simulink model "Engine_MC_Wit_System1"  (R2014b)
settings: Solver=ode15s  StartTime=0.0  StopTime=100  RelTol=1e-3
undefined symbols (not defined in the file): sigbuilder_block
libraries: fl_lib x19, nesl_utility x9, sdl_lib x4, simulink x4
settings Model: Creator=wnursilo  LastModifiedBy=wnursilo
settings SolverCC: ZeroCrossAlgorithm=Adaptive
settings SimscapeCC: SimscapeLogType=local  SimscapeLogLimitData=off

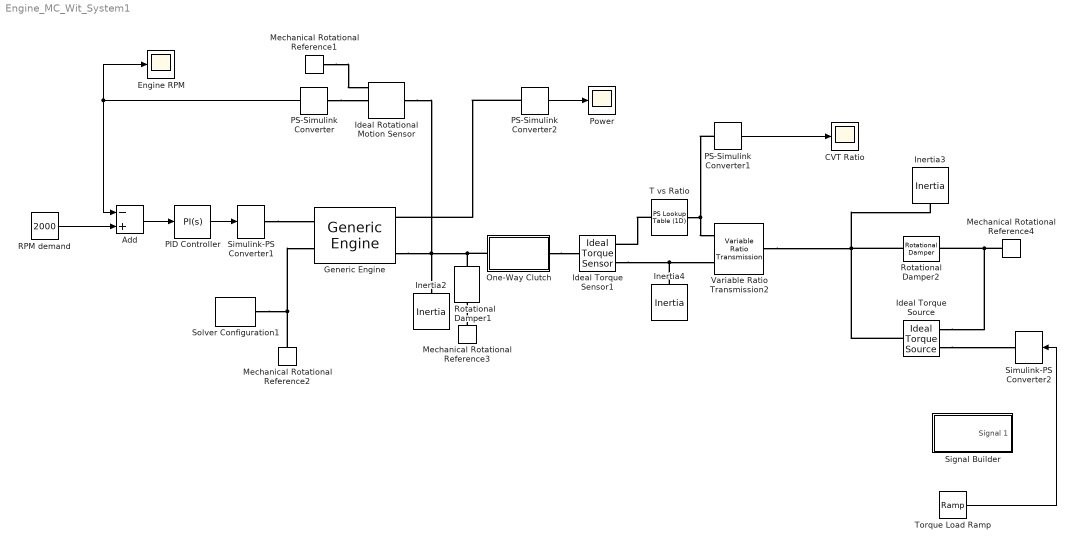
== system Engine_MC_Wit_System1 ==
  Add : Sum  Inputs=-+
  CVT Ratio : Scope
      settings: YMin=3  YMax=11
  Engine RPM : Scope
      settings: YMin=750  YMax=2750
  Generic Engine : sdl_lib/Engines/Generic Engine  model_parameterization=1  engine_type=1  P_max=8300 W  w_P_max=8500 rpm  w_max=9000 rpm  w_min=500 rpm  w_tab=[ 500 1000 2e+3 3e+3 4e+3 5e+3 6e+3 7e+3 ] rpm  trq_tab=[ 380 380 380 380 350 280 200 80 ] N*m  pwr_tab=[ 2e+4 4e+4 7.8e+4 1.2e+5 1.45e+5 1.48e+5 1.25e+5 6e+4 ] W  interp_method=1  model_inertia=0  inertia=1 kg*m^2  initial_velocity=800 rpm  model_time_constant=0  time_constant=0.2 s  T0=0  w_thr=100 rpm  idle_speed=0  idle_speed_reference=1000 rpm  tau_controller=0.1 s  idle_w_thr=10 rpm  fc_model=1  fc_per_rev=25 mg/rev  displaced_volume=400 cm^3  rev_per_cycle=2  fc_w_tab=[ 1000 2e+3 3e+3 4e+3 5e+3 6e+3 ] rpm  fc_trq_tab=[ 0 80 160 200 240 320 360 400 ] N*m  fc_tab=[ 0.5 0.9 1.4 1.6 1.9 2.7 3.4 4.4; 1 1.7 2.7 3.1 3.6 5 6 7.4; 1.4 2.7 4 4.8 5.6 7.5 8.5 10.5; 2 3.6 5.8 6.7 8 10.4 11.7 13.3; 2.5 4.8 7.9 9.4 10.8 14 16.2 18.6; 3.1 6 10.3 11.9 13.8 18.4 22 26.5 ] g/s  bmep_tab=[ 0 250 500 625 750 1000 1.15e+3 1.25e+3 ] kPa  bsfc_tab=[ 410 380 300 280 270 290 320 380; 410 370 290 270 260 270 285 320; 415 380 290 275 265 270 270 300; 420 390 310 290 285 280 280 285; 430 410 340 320 310 300 310 320; 450 430 370 340 330 330 350 380 ] g/hr/kW  fc_interp_method=1
  Ideal Rotational Motion Sensor : fl_lib/Mechanical/Mechanical Sensors/Ideal Rotational Motion Sensor  offset=0 rad
  Ideal Torque Sensor1 : fl_lib/Mechanical/Mechanical Sensors/Ideal Torque Sensor
  Ideal Torque Source : fl_lib/Mechanical/Mechanical Sources/Ideal Torque Source
  Inertia2 : fl_lib/Mechanical/Rotational Elements/Inertia  inertia=HEV_Param.ICE.Shaft_Inertia kg*m^2  w_specify=on  w_priority=High  w=800 rpm  t_specify=off  t_priority=High  t=0 N*m
  Inertia3 : fl_lib/Mechanical/Rotational Elements/Inertia  inertia=HEV_Param.ICE.Shaft_Inertia kg*m^2  w_specify=on  w_priority=Low  w=0 rad/s  t_specify=off  t_priority=High  t=0 N*m
      settings: LogSimulationData=on
  Inertia4 : fl_lib/Mechanical/Rotational Elements/Inertia  inertia=HEV_Param.ICE.Shaft_Inertia kg*m^2  w_specify=on  w_priority=Low  w=0 rpm  t_specify=off  t_priority=High  t=0 N*m
  Mechanical Rotational Reference{1..4} (4 alike) : fl_lib/Mechanical/Rotational Elements/Mechanical Rotational Reference
  One-Way Clutch : Subsystem
  PID Controller : simulink/Continuous/PID Controller  Controller=PI  TimeDomain=Continuous-time  SampleTime=-1  IntegratorMethod=Forward Euler  FilterMethod=Forward Euler  Form=Parallel  P=10  I=1  D=0  N=100  InitialConditionSource=internal  InitialConditionForIntegrator=0  InitialConditionForFilter=0  ExternalReset=none  LimitOutput=off  UpperSaturationLimit=inf  LowerSaturationLimit=-inf  LinearizeAsGain=on  AntiWindupMode=none  Kb=1  TrackingMode=off  Kt=1  PParamMin=[]  PParamMax=[]  IParamMin=[]  IParamMax=[]  DParamMin=[]  DParamMax=[]  NParamMin=[]  NParamMax=[]  KbParamMin=[]  KbParamMax=[]  KtParamMin=[]  KtParamMax=[]  POutMin=[]  POutMax=[]  IOutMin=[]  IOutMax=[]  DOutMin=[]  DOutMax=[]  NOutMin=[]  NOutMax=[]  KbOutMin=[]  KbOutMax=[]  KtOutMin=[]  KtOutMax=[]  IntegratorOutMin=[]  IntegratorOutMax=[]  FilterOutMin=[]  FilterOutMax=[]  SumOutMin=[]  SumOutMax=[]  SumI1OutMin=[]  SumI1OutMax=[]  SumI2OutMin=[]  SumI2OutMax=[]  SumI3OutMin=[]  SumI3OutMax=[]  SumDOutMin=[]  SumDOutMax=[]  SaturationOutMin=[]  SaturationOutMax=[]  IntegratorContinuousStateAttributes=''  IntegratorStateMustResolveToSignalObject=off  IntegratorRTWStateStorageClass=Auto  FilterContinuousStateAttributes=''  FilterStateMustResolveToSignalObject=off  FilterRTWStateStorageClass=Auto  DifferentiatorICPrevScaledInput=0  DifferentiatorOutMin=[]  DifferentiatorOutMax=[]  UseFilter=on
  PS-Simulink Converter : nesl_utility/PS-Simulink Converter  PhysicalDomain=network_engine_domain  SubClassName=ps_output  LeftPortType=input  RightPortType=output  PseudoPeriodic=off  Frequencies=[]  Unit=rpm  AffineConversion=off
  PS-Simulink Converter1 : nesl_utility/PS-Simulink Converter  PhysicalDomain=network_engine_domain  SubClassName=ps_output  LeftPortType=input  RightPortType=output  PseudoPeriodic=off  Frequencies=[]  Unit=1  AffineConversion=off
  PS-Simulink Converter2 : nesl_utility/PS-Simulink Converter  PhysicalDomain=network_engine_domain  SubClassName=ps_output  LeftPortType=input  RightPortType=output  PseudoPeriodic=off  Frequencies=[]  Unit=1  AffineConversion=off
  Power : Scope
      settings: YMin=5250  YMax=7500  SaveName=ScopeData3
  RPM demand : Constant  Value=2000
  Rotational Damper1 : fl_lib/Mechanical/Rotational Elements/Rotational Damper  D=0.01 N*m/(rad/s)  w_specify=off  w_priority=High  w=0 rad/s  t_specify=off  t_priority=High  t=0 N*m
  Rotational Damper2 : fl_lib/Mechanical/Rotational Elements/Rotational Damper  D=0.001 N*m/(rad/s)  w_specify=off  w_priority=High  w=0 rad/s  t_specify=off  t_priority=High  t=0 N*m
  Signal Builder : Subsystem  Tag=STV Subsys  LoadFcn=sigbuilder_block('load');  StartFcn=sigbuilder_block('start');  StopFcn=sigbuilder_block('stop');  ClipboardFcn=sigbuilder_block('clipboard');  mask(Sigbuilder block){}
      mask help: Simulink:masks:SigbuilderBlock_MD
      mask init:
      | if ~strcmp(get_param(bdroot(gcbh),'SimulationStatus'),'stopped') tuvar = sigbuilder_block('maskInit'); end
      settings: CopyFcn=sigbuilder_block('copy');  DeleteFcn=sigbuilder_block('delete');  ModelCloseFcn=sigbuilder_block('modelClose');  PreSaveFcn=sigbuilder_block('preSave');  PauseFcn=sigbuilder_block('pause');  ContinueFcn=sigbuilder_block('continue');  NameChangeFcn=sigbuilder_block('namechange');  OpenFcn=sigbuilder_block('open',[437.25 199.5 550.5 399.75 ]);  CloseFcn=sigbuilder_block('close');
      mask Display: plot(0, 0, 100, 100,[2, 2, 32, 32, 2], [68, 8, 8, 68, 68],[32, 2], [38, 38], [32, 19, 2],[53, 60, 44], [32, 17, 17, 2],[16, 16, 31, 31]);txt = getActiveGroup(gcbh);text(2, 100, txt,'verticalAlignment', 'top');
  Simulink-PS Converter1 : nesl_utility/Simulink-PS Converter  PhysicalDomain=network_engine_domain  SubClassName=ps_input  LeftPortType=input  RightPortType=output  PseudoPeriodic=off  Frequencies=[]  NoiseDistribution=none  NoiseParameters=[]  Unit=1  AffineConversion=off  InputFiltering=on  SimscapeFilterOrder=1  InputFilterTimeConstant=0.001  UdotUserProvided=1
  Simulink-PS Converter2 : nesl_utility/Simulink-PS Converter  PhysicalDomain=network_engine_domain  SubClassName=ps_input  LeftPortType=input  RightPortType=output  PseudoPeriodic=off  Frequencies=[]  NoiseDistribution=none  NoiseParameters=[]  Unit=1  AffineConversion=off  InputFiltering=off  SimscapeFilterOrder=1  InputFilterTimeConstant=0.001  UdotUserProvided=1
  Solver Configuration1 : nesl_utility/Solver Configuration  PhysicalDomain=network_engine_domain  SubClassName=solver  LeftPortType=input  RightPortType=generic  Accelerate=off  Tones=[]  Harmonics=[]  SimulateNoise=off  Profile=off  UseLocalSampling=off  EnableSwitchedLinearOptims=on  FrequencyDomain=off  UseCCode=off  RelTol=0.001  AbsTol=1e-06  MinStep=1e-09  ToWorkspace=off  DoDC=off  ResidualTolerance=1e-09  UseLocalSolver=off  LocalSolverChoice=NE_BACKWARD_EULER_ADVANCER  LocalSolverSampleTime=0.001  DoFixedCost=off  MaxNonlinIter=3  MaxModeIter=2  LinearAlgebra=Sparse  DelaysMemoryBudget=1024  AutomaticFiltering=on  FilteringTimeConstant=0.001
  T vs Ratio : fl_lib/Physical Signals/Lookup Tables/PS Lookup Table (1D)  x_t="[1e3, 100,  80, 60, 40, 20, 10, 8, 6, 4, 2, 0]"  y_t=[10, 10, 8, 6, 4, 2, 1, 0.8, 0.6, 0.4, 0.2, 0.2]  interp_method=1  extrap_method=2
  Torque Load Ramp : simulink/Sources/Ramp  slope=-10  start=2  X0=0
  Variable Ratio Transmission2 : sdl_lib/Couplings & Drives/Variable Ratio Transmission  rotation_direction=1  kp=3e+5 N*m/rad  kv=100 N*m/(rad/s)  initial_torque=0 N*m  losses_model=1  efficiency=0.8  mu_visc=[ 0 0 ] N*m/(rad/s)  w_thr=0.01 rad/s
  wires:
  RPM demand/1 -> Add/2
  PS-Simulink Converter/1 -> Engine RPM/1, Add/1
  Add/1 -> PID Controller/1
  PID Controller/1 -> Simulink-PS Converter1/1
  Torque Load Ramp/1 -> Simulink-PS Converter2/1
  PS-Simulink Converter1/1 -> CVT Ratio/1
  PS-Simulink Converter2/1 -> Power/1
  connections:
  Mechanical Rotational Reference2/LConn1 -- Solver Configuration1/RConn1 -- Generic Engine/LConn2
  Generic Engine/RConn3 -- One-Way Clutch/LConn1 -- Rotational Damper1/LConn1 -- Ideal Rotational Motion Sensor/LConn1 -- Inertia2/LConn1
  Simulink-PS Converter1/RConn1 -- Generic Engine/LConn1
  Mechanical Rotational Reference3/LConn1 -- Rotational Damper1/RConn1
  Rotational Damper2/LConn1 -- Ideal Torque Source/LConn1 -- Inertia3/LConn1 -- Variable Ratio Transmission2/RConn1
  Mechanical Rotational Reference4/LConn1 -- Ideal Torque Source/RConn2 -- Rotational Damper2/RConn1
  One-Way Clutch/RConn1 -- Ideal Torque Sensor1/LConn1
  Ideal Torque Sensor1/RConn1 -- Inertia4/LConn1 -- Variable Ratio Transmission2/LConn2
  T vs Ratio/LConn1 -- Ideal Torque Sensor1/RConn2
  T vs Ratio/RConn1 -- Variable Ratio Transmission2/LConn1 -- PS-Simulink Converter1/LConn1
  PS-Simulink Converter/LConn1 -- Ideal Rotational Motion Sensor/RConn2
  Mechanical Rotational Reference1/LConn1 -- Ideal Rotational Motion Sensor/RConn1
  Ideal Torque Source/RConn1 -- Simulink-PS Converter2/RConn1
  PS-Simulink Converter2/LConn1 -- Generic Engine/RConn1

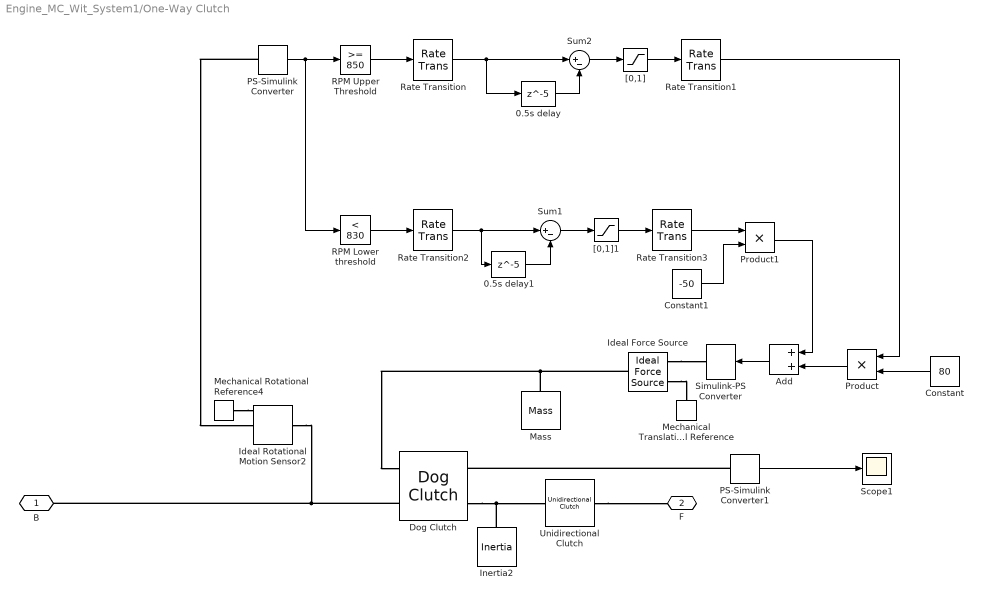
== system Engine_MC_Wit_System1/One-Way Clutch ==
  0.5s delay : Delay  DelayLength=5  SampleTime=0.01
  0.5s delay1 : Delay  DelayLength=5  SampleTime=0.01
  Add : Sum
  Constant : Constant  Value=80
  Constant1 : Constant  Value=-50
  Dog Clutch : sdl_lib/Clutches/Dog Clutch  model=1  max_torque=10000 N*m  n_teeth=6  clutch_backlash=10 deg  tooth_height=10 mm  radius=50 mm  back_stop=1  ring_hub_gap=3 mm  clutch_stiffness=1e+7 N*m/rad  clutch_damping=100 N*m/(rad/s)  transl_stiffness=1e+6 N/m  transl_damping=100000 N/(m/s)  visc_fric_transl=10 N/(m/s)  fric_coeff=0.05  direction=1  engagement_velocity=Inf rad/s  engagement_overlap=3 mm  initial_state_engaged=0  init_pos=0 mm  init_rel_angle=0 deg
  Ideal Force Source : fl_lib/Mechanical/Mechanical Sources/Ideal Force Source
  Ideal Rotational Motion Sensor2 : fl_lib/Mechanical/Mechanical Sensors/Ideal Rotational Motion Sensor  offset=0 rad
  Inertia2 : fl_lib/Mechanical/Rotational Elements/Inertia  inertia=0.001 kg*m^2  w_specify=on  w_priority=Low  w=0 rpm  t_specify=off  t_priority=High  t=0 N*m
  Mass : fl_lib/Mechanical/Translational Elements/Mass  mass=0.1 kg  v_specify=on  v_priority=Low  v=0 m/s  f_specify=off  f_priority=High  f=0 N
  Mechanical Rotational Reference4 : fl_lib/Mechanical/Rotational Elements/Mechanical Rotational Reference
  Mechanical Translational Reference : fl_lib/Mechanical/Translational Elements/Mechanical Translational Reference
  PS-Simulink Converter : nesl_utility/PS-Simulink Converter  PhysicalDomain=network_engine_domain  SubClassName=ps_output  LeftPortType=input  RightPortType=output  PseudoPeriodic=off  Frequencies=[]  Unit=rpm  AffineConversion=off
  PS-Simulink Converter1 : nesl_utility/PS-Simulink Converter  PhysicalDomain=network_engine_domain  SubClassName=ps_output  LeftPortType=input  RightPortType=output  PseudoPeriodic=off  Frequencies=[]  Unit=mm  AffineConversion=off
  Product : Product
  Product1 : Product
  RPM Lower threshold : simulink/Logic and Bit Operations/Compare To Constant  relop=<  const=830  OutDataTypeStr=uint8  ZeroCross=off
  RPM Upper Threshold : simulink/Logic and Bit Operations/Compare To Constant  relop=>=  const=850  OutDataTypeStr=uint8  ZeroCross=off
  Rate Transition : RateTransition  OutPortSampleTime=0.01
  Rate Transition1 : RateTransition  OutPortSampleTime=0.001
  Rate Transition2 : RateTransition  OutPortSampleTime=0.01
  Rate Transition3 : RateTransition  OutPortSampleTime=0.001
  Scope1 : Scope
      settings: YMin=-2.5  YMax=15  SaveName=ScopeData2
  Simulink-PS Converter : nesl_utility/Simulink-PS Converter  PhysicalDomain=network_engine_domain  SubClassName=ps_input  LeftPortType=input  RightPortType=output  PseudoPeriodic=off  Frequencies=[]  NoiseDistribution=none  NoiseParameters=[]  Unit=1  AffineConversion=off  InputFiltering=off  SimscapeFilterOrder=1  InputFilterTimeConstant=0.001  UdotUserProvided=1
  Sum1 : Sum  Inputs=|+-  SaturateOnIntegerOverflow=on  InputSameDT=on  OutDataTypeStr=Inherit: Same as first input
  Sum2 : Sum  Inputs=|+-  SaturateOnIntegerOverflow=on  InputSameDT=on  OutDataTypeStr=Inherit: Same as first input
  Unidirectional Clutch : sdl_lib/Clutches/Unidirectional Clutch  transmission_direction=1  initial_state_locked=0
  "[0,1]" : Saturate  UpperLimit=1  LowerLimit=0  OutDataTypeStr=double
  "[0,1]1" : Saturate  UpperLimit=1  LowerLimit=0  OutDataTypeStr=double
  B : PMIOPort  Port=1  Side=Left
  F : PMIOPort  Port=2  Side=Right
  wires:
  PS-Simulink Converter/1 -> RPM Lower threshold/1, RPM Upper Threshold/1
  Rate Transition/1 -> 0.5s delay/1, Sum2/1
  Sum2/1 -> "[0,1]"/1
  0.5s delay/1 -> Sum2/2
  RPM Upper Threshold/1 -> Rate Transition/1
  "[0,1]"/1 -> Rate Transition1/1
  Rate Transition1/1 -> Product/1
  PS-Simulink Converter1/1 -> Scope1/1
  Constant/1 -> Product/2
  RPM Lower threshold/1 -> Rate Transition2/1
  Rate Transition2/1 -> 0.5s delay1/1, Sum1/1
  Sum1/1 -> "[0,1]1"/1
  0.5s delay1/1 -> Sum1/2
  "[0,1]1"/1 -> Rate Transition3/1
  Rate Transition3/1 -> Product1/1
  Constant1/1 -> Product1/2
  Add/1 -> Simulink-PS Converter/1
  Product/1 -> Add/2
  Product1/1 -> Add/1
  connections:
  Unidirectional Clutch/RConn1 -- F/RConn1
  Dog Clutch/RConn2 -- Unidirectional Clutch/LConn1 -- Inertia2/LConn1
  Mechanical Rotational Reference4/LConn1 -- Ideal Rotational Motion Sensor2/RConn1
  Ideal Rotational Motion Sensor2/LConn1 -- Dog Clutch/LConn2 -- B/RConn1
  PS-Simulink Converter/LConn1 -- Ideal Rotational Motion Sensor2/RConn2
  Ideal Force Source/RConn1 -- Simulink-PS Converter/RConn1
  Ideal Force Source/LConn1 -- Dog Clutch/LConn1 -- Mass/LConn1
  Ideal Force Source/RConn2 -- Mechanical Translational Reference/LConn1
  PS-Simulink Converter1/LConn1 -- Dog Clutch/RConn1

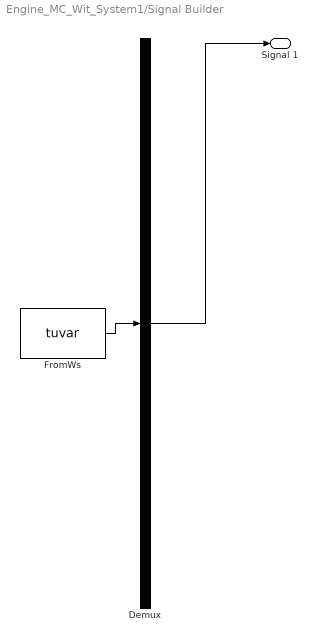
== system Engine_MC_Wit_System1/Signal Builder ==
  Demux : Demux  Tag=STV Demux  Outputs=1
  FromWs : FromWorkspace  Tag=STV FromWs  VariableName=tuvar  SampleTime=0
      SigBuilderData=|
      | common.afterFinalStr = 'Extrapolate'
      | common.sampleTime = 0
      | dataSet.timeRange = [0 10]
      | dataSet.name = 'Group 1'
      | sbobj.Groups.Name = 'Group 1'
      | sbobj.Groups.Signals.Name = 'Signal 1'
      | sbobj.Groups.Signals.XData = [0 1 6 8.02 8.02 10]
      | sbobj.Groups.Signals.YData = [0 0 -10 -10 0 0]
  Signal 1 : Outport  Tag=STV Outport
  wires:
  FromWs/1 -> Demux/1
  Demux/1 -> Signal 1/1
